simulink model "trzzy_kanaly_serial_real"  (R2025b)
settings: Solver=VariableStepAuto  StartTime=0.0  StopTime=0.5  RelTol=1e-3
undefined symbols (not defined in the file or in its folder): c, dspblkCoreblockFVToolHelper, gcbh, sfvc784, xck26
libraries: hdlBasic x68, simulink x5, hdlUtilities x4, vmcUtilities x1
settings Model: Creator=janek  LastModifiedBy=janek

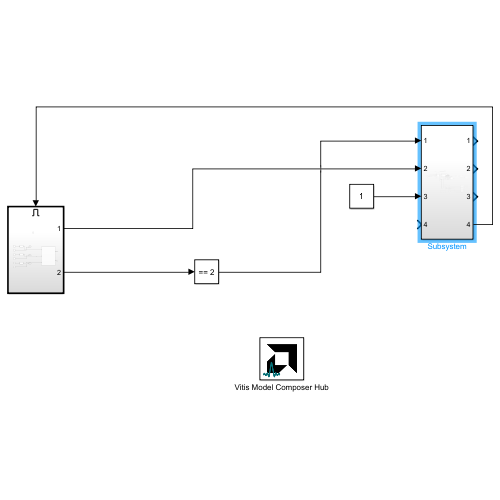
[thumbnail: Simulink's stored preview of the top-level diagram]
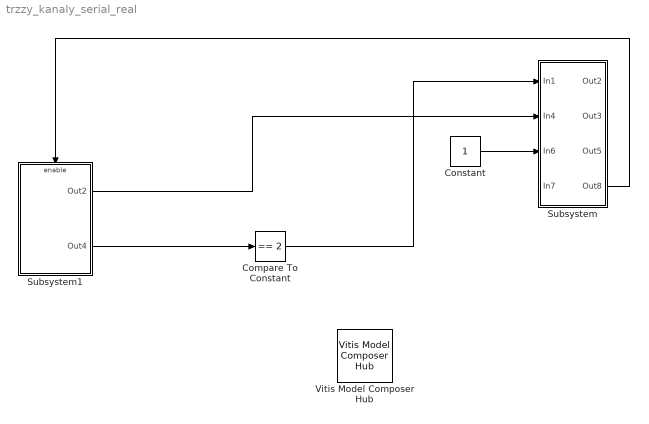
== system trzzy_kanaly_serial_real ==
  Compare To Constant : simulink/Logic and Bit Operations/Compare To Constant  relop===  const=2  OutDataTypeStr=boolean
  Constant : Constant
  Subsystem : Subsystem
  Subsystem1 : Subsystem
  Vitis Model Composer Hub : vmcUtilities/Vitis Model Composer Hub  Tag=genX  CodeGeneration=off  SubsystemName=Subsystem  CompilationType=HDLCompilation  ExportTypeV2=IP Catalog  StartColumn=1  NumberOfColumns=1  TargetDirectory=./netlist  exportDesign=off  analyzeDesign=off  validateDesignOnHw=off  ExportType=AI Engines  IpVendor=xilinx.com  IpLibrary=hls  IpVersion=1.0  IpHWLanguage=Verilog  AieCompilerOptions={}  AieSimulatorOptions={}  CreateTestbench=off  TestbenchStackSize=10  RunRtlSim=off  RunCSim=off  RunAieSim=off  AieSimTimeout=50000  RunAieSimProfiling=off  LaunchVitisAnalyzer=off  PlotOutput=off  RunX86Sim=off  X86SimTimeout=10  GenHwImage=off  GenLibadfXo=on  GenHwValidationCode=off  PlatformType=Not Specified  HwSystemType=Baremetal  HwValidationTarget=hw  ProjDevice=Kria KR260 Robotics Starter Kit SOM (xck26-sfvc784-2LV-c)  ProjDevicePart=xck26-sfvc784-2LV-c  AIEType=None  SamplePeriod=-1  ClockFrequency=200  DataPathParallelism=1  xilinxfamily=zynquplus  part=xck26  speed=-2LV-c  package=sfvc784  directory=./netlist\ip\Subsystem\src  testbench=off  incr_netlist=off  synthesis_tool=Vivado  clock_wrapper=Clock Enables  dbl_ovrd=According to Block Masks  dcm_input_clock_period=10  sysclk_period=40  simulink_period=1/81000  eval_field=0  LogFileName=''  NThreads=4
  wires:
  Compare To Constant/1 -> Subsystem/1(In1)
  Constant/1 -> Subsystem/3(In6)
  Subsystem1/2(Out4) -> Compare To Constant/1
  Subsystem/4(Out8) -> Subsystem1/Enable
  Subsystem1/1(Out2) -> Subsystem/2(In4)

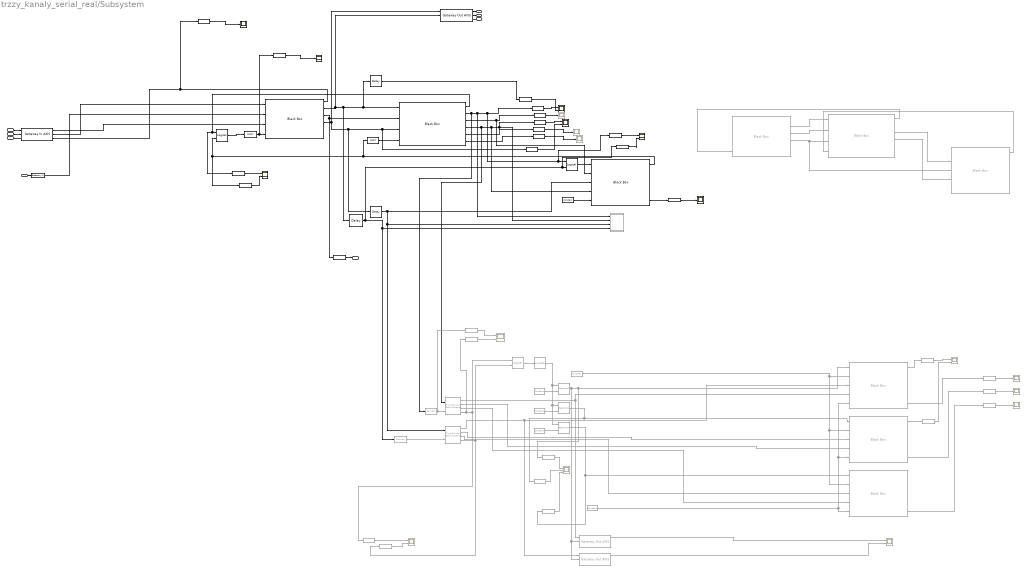
== system trzzy_kanaly_serial_real/Subsystem ==
  In1 : Inport
  In4 : Inport  Port=2
  In6 : Inport  Port=3
  In7 : Inport  Port=4
  Assert : hdlBasic/Assert  assert_type=on  type_source=Explicitly  gui_display_data_type=Fixed-point  arith_type=Unsigned  n_bits=1  bin_pt=0  preci_type=Single  exp_width=8  frac_width=24  assert_rate=on  rate_source=Explicitly  period=1/81000  output_port=on  XmcBlockStatus=1  maskContainerNames=group1  block_type=assert  block_config=sysgen:assert_config  block_width=609  block_height=900
  Assert1 : hdlBasic/Assert  assert_type=on  type_source=Explicitly  gui_display_data_type=Fixed-point  arith_type=Unsigned  n_bits=1  bin_pt=0  preci_type=Single  exp_width=8  frac_width=24  assert_rate=on  rate_source=Explicitly  period=1/81000  output_port=on  XmcBlockStatus=1  maskContainerNames=group1  block_type=assert  block_config=sysgen:assert_config  block_width=609  block_height=900
  Black Box : hdlBasic/Black Box  init_code=fir_compiler_0_wrapper_config  sim_method=Vivado Simulator  verbose=off  XmcBlockStatus=1  maskContainerNames=group1  block_type=blackbox2  block_config=sysgen:black_box_config
  Black Box1 : hdlBasic/Black Box  init_code=fir_compiler_1_wrapper_config  sim_method=Vivado Simulator  verbose=off  XmcBlockStatus=1  maskContainerNames=group1  block_type=blackbox2  block_config=sysgen:black_box_config
  Black Box2 : hdlBasic/Black Box  Commented=on  init_code=fir_compiler_0_wrapper_config  sim_method=Vivado Simulator  verbose=off  XmcBlockStatus=1  maskContainerNames=group1  block_type=blackbox2  block_config=sysgen:black_box_config
  Black Box3 : hdlBasic/Black Box  Commented=on  init_code=fir_compiler_1_wrapper_config  sim_method=Vivado Simulator  verbose=off  XmcBlockStatus=1  maskContainerNames=group1  block_type=blackbox2  block_config=sysgen:black_box_config
  Black Box{4,7..9} (4 alike) : hdlBasic/Black Box  Commented=on  init_code=cordic_0_wrapper_config  sim_method=Vivado Simulator  verbose=off  XmcBlockStatus=1  maskContainerNames=group1  block_type=blackbox2  block_config=sysgen:black_box_config
  Black Box5 : hdlBasic/Black Box  init_code=cordic_0_wrapper_config  sim_method=Vivado Simulator  verbose=off  XmcBlockStatus=1  maskContainerNames=group1  block_type=blackbox2  block_config=sysgen:black_box_config
  Constant : hdlBasic/Constant  const=1.0  gui_display_data_type=Boolean  arith_type=Boolean  n_bits=16  bin_pt=14  preci_type=Single  exp_width=8  frac_width=24  explicit_period=off  period=1  XmcBlockStatus=1  maskContainerNames=tabcontainer1  block_type=constant  block_config=sysgen:Constant_config
  Constant3 : hdlBasic/Constant  Commented=on  const=0  gui_display_data_type=Fixed-point  arith_type=Signed (2's comp)  n_bits=2  bin_pt=0  preci_type=Single  exp_width=8  frac_width=24  explicit_period=off  period=1  XmcBlockStatus=1  maskContainerNames=tabcontainer1  block_type=constant  block_config=sysgen:Constant_config
  Constant4 : hdlBasic/Constant  Commented=on  const=1.0  gui_display_data_type=Fixed-point  arith_type=Unsigned  n_bits=2  bin_pt=0  preci_type=Single  exp_width=8  frac_width=24  explicit_period=off  period=1  XmcBlockStatus=1  maskContainerNames=tabcontainer1  block_type=constant  block_config=sysgen:Constant_config
  Constant5 : hdlBasic/Constant  Commented=on  const=2  gui_display_data_type=Fixed-point  arith_type=Unsigned  n_bits=2  bin_pt=0  preci_type=Single  exp_width=8  frac_width=24  explicit_period=off  period=1  XmcBlockStatus=1  maskContainerNames=tabcontainer1  block_type=constant  block_config=sysgen:Constant_config
  Constant6 : hdlBasic/Constant  Commented=on  const=1.0  gui_display_data_type=Boolean  arith_type=Boolean  n_bits=16  bin_pt=14  preci_type=Single  exp_width=8  frac_width=24  explicit_period=off  period=1  XmcBlockStatus=1  maskContainerNames=tabcontainer1  block_type=constant  block_config=sysgen:Constant_config
  Constant7 : hdlBasic/Constant  Commented=on  const=0  gui_display_data_type=Boolean  arith_type=Boolean  n_bits=2  bin_pt=0  preci_type=Single  exp_width=8  frac_width=24  explicit_period=off  period=1  XmcBlockStatus=1  maskContainerNames=tabcontainer1  block_type=constant  block_config=sysgen:Constant_config
  Convert5 : hdlBasic/Convert  Commented=on  gui_display_data_type=Boolean  arith_type=Boolean  n_bits=16  bin_pt=14  float_type=Single  exp_bits=8  fraction_bits=24  quantization=Truncate  overflow=Wrap  en=off  latency=0  pipeline=off  XmcBlockStatus=1  maskContainerNames=group2  block_type=convert  block_config=sysgen:Convert_config  block_width=595  block_height=885
  Convert6 : hdlBasic/Convert  Commented=on  gui_display_data_type=Boolean  arith_type=Boolean  n_bits=16  bin_pt=14  float_type=Single  exp_bits=8  fraction_bits=24  quantization=Truncate  overflow=Wrap  en=off  latency=0  pipeline=off  XmcBlockStatus=1  maskContainerNames=group2  block_type=convert  block_config=sysgen:Convert_config  block_width=595  block_height=885
  Counter : hdlBasic/Counter  Commented=on  cnt_type=Count limited  cnt_to=2  operation=Up  start_count=0  cnt_by_val=1  arith_type=Unsigned  n_bits=2  bin_pt=0  load_pin=off  rst=off  en=on  explicit_period=Explicit  period=1/27000  use_behavioral_HDL=off  implementation=Fabric  XmcBlockStatus=1  maskContainerNames=group1  block_type=counter  block_config=sysgen:Counter_config  block_width=531  block_height=1023
  Delay : hdlBasic/Delay  rst=off  en=off  latency=30  reg_retiming=off  XmcBlockStatus=1  maskContainerNames=group1  block_type=delay  block_config=sysgen:Delay_config
  Delay1 : hdlBasic/Delay  rst=off  en=off  latency=30  reg_retiming=off  XmcBlockStatus=1  maskContainerNames=group1  block_type=delay  block_config=sysgen:Delay_config
  Delay2 : hdlBasic/Delay  rst=off  en=off  latency=30  reg_retiming=off  XmcBlockStatus=1  maskContainerNames=group1  block_type=delay  block_config=sysgen:Delay_config
  Gateway In : hdlBasic/Gateway In  gui_display_data_type=Boolean  arith_type=Boolean  n_bits=16  bin_pt=14  preci_type=Single  exp_width=8  frac_width=24  rows=1  columns=1  quantization="Round  (unbiased: +/- Inf)"  overflow=Saturate  period=1/81000  UseAsADC=off  ADCChannel='1'  interface=None  automatic_assignment=on  address_offset=hex2dec('00')  intf_name=''  intf_description=''  default_value=0  timing_constraint=None  locs_specified=off  LOCs={}  io_standard={}  inherit_from_input=off  hdl_port=on  XmcBlockStatus=1  maskContainerNames=group4  block_type=gatewayin  block_config=sysgen:gateway_in_config  block_width_w=590  block_height_w=620  block_width=640  block_height=850
  Gateway In AXIS : hdlUtilities/Gateway In AXIS  gui_display_data_type=Fixed-point  arith_type=Signed (2's comp)  n_bits=16  bin_pt=14  preci_type=Custom  exp_width=16  frac_width=24  quantization="Round  (unbiased: +/- Inf)"  overflow=Wrap  bool_to_boolean=off  OutSampleTime=1/81000  block_type=gatewayinaxi  XmcBlockStatus=1
  Gateway Out{,1..14} (15 alike) : hdlBasic/Gateway Out  inherit_from_input=off  bool_to_boolean=off  hdl_port=on  rows=1  columns=1  UseAsDAC=off  DACChannel='1'  interface=None  automatic_assignment=on  address_offset=hex2dec('00')  intf_name=''  intf_description=''  timing_constraint=None  locs_specified=off  LOCs={}  io_standard={}  XmcBlockStatus=1  maskContainerNames=group4  block_type=gatewayout  block_config=sysgen:gateway_out_config  block_width_w=590  block_height_w=620  block_width=620  block_height=750
  Gateway Out AXIS : hdlUtilities/Gateway Out AXIS  mask_sample_period=1/81000  bool_to_boolean=off  block_type=gatewayoutaxi
  Gateway Out AXIS1 : hdlUtilities/Gateway Out AXIS  Commented=on  mask_sample_period=1/27000  bool_to_boolean=off  block_type=gatewayoutaxi
  Gateway Out AXIS2 : hdlUtilities/Gateway Out AXIS  Commented=on  mask_sample_period=1/27000  bool_to_boolean=off  block_type=gatewayoutaxi
  Gateway Out{18..29} (12 alike) : hdlBasic/Gateway Out  Commented=on  inherit_from_input=off  bool_to_boolean=off  hdl_port=on  rows=1  columns=1  UseAsDAC=off  DACChannel='1'  interface=None  automatic_assignment=on  address_offset=hex2dec('00')  intf_name=''  intf_description=''  timing_constraint=None  locs_specified=off  LOCs={}  io_standard={}  XmcBlockStatus=1  maskContainerNames=group4  block_type=gatewayout  block_config=sysgen:gateway_out_config  block_width_w=590  block_height_w=620  block_width=620  block_height=750
  Logical : hdlBasic/Logical  logical_function=AND  inputs=2  en=off  latency=0  precision=Full  arith_type=Unsigned  n_bits=16  bin_pt=0  align_bp=on  overflow=[]  quantization=[]  XmcBlockStatus=1  maskContainerNames=tabcontainer1  block_type=logical  block_config=sysgen:Logical_config
  Logical1 : hdlBasic/Logical  logical_function=AND  inputs=2  en=off  latency=0  precision=Full  arith_type=Unsigned  n_bits=16  bin_pt=0  align_bp=on  overflow=[]  quantization=[]  XmcBlockStatus=1  maskContainerNames=tabcontainer1  block_type=logical  block_config=sysgen:Logical_config
  Logical2 : hdlBasic/Logical  Commented=on  logical_function=AND  inputs=2  en=off  latency=0  precision=Full  arith_type=Unsigned  n_bits=16  bin_pt=0  align_bp=on  overflow=[]  quantization=[]  XmcBlockStatus=1  maskContainerNames=tabcontainer1  block_type=logical  block_config=sysgen:Logical_config
  Relational : hdlBasic/Relational  Commented=on  mode=a=b  op_type=Bool  en=off  latency=0  XmcBlockStatus=1  maskContainerNames=tabcontainer1  block_type=relational  block_config=sysgen:Relational_config
  Relational1 : hdlBasic/Relational  Commented=on  mode=a=b  op_type=Bool  en=off  latency=0  XmcBlockStatus=1  maskContainerNames=tabcontainer1  block_type=relational  block_config=sysgen:Relational_config
  Relational2 : hdlBasic/Relational  Commented=on  mode=a=b  op_type=Bool  en=off  latency=0  XmcBlockStatus=1  maskContainerNames=tabcontainer1  block_type=relational  block_config=sysgen:Relational_config
  Scope{,1,6..7} (4 alike) : Scope  NumInputPorts=2
      Scope settings: ActiveDisplayYMinimum=-0.12499999999999997  ActiveDisplayYMaximum=1.125
      Scope1 settings: ActiveDisplayYMinimum=-1  ActiveDisplayYMaximum=1
      Scope6 settings: ActiveDisplayYMinimum=-0.12499999999999997  ActiveDisplayYMaximum=1.125  DataLoggingVariableName=ScopeData6
      Scope7 settings: ActiveDisplayYMinimum=-0.12499999999999997  ActiveDisplayYMaximum=1.125  DataLoggingVariableName=ScopeData7
  Scope{2..4,15..17} (6 alike) : Scope  Commented=on
      Scope15 settings: ActiveDisplayYMinimum=-3.2137215999999993E+7  ActiveDisplayYMaximum=2.89234944E+8  DataLoggingVariableName=ScopeData15
      Scope16 settings: ActiveDisplayYMinimum=-3.2137215999999993E+7  ActiveDisplayYMaximum=2.89234944E+8  DataLoggingVariableName=ScopeData16
      Scope17 settings: ActiveDisplayYMinimum=-3.2137215999999993E+7  ActiveDisplayYMaximum=2.89234944E+8  DataLoggingVariableName=ScopeData17
      Scope2 settings: ActiveDisplayYMinimum=-1  ActiveDisplayYMaximum=1  DataLoggingVariableName=ScopeData2
      Scope3 settings: ActiveDisplayYMinimum=-1  ActiveDisplayYMaximum=1  DataLoggingVariableName=ScopeData3
      Scope4 settings: ActiveDisplayYMinimum=-0.12499999999999997  ActiveDisplayYMaximum=1.125  DataLoggingVariableName=ScopeData4
  Scope{18..21} (4 alike) : Scope  Commented=on  NumInputPorts=2
      Scope18 settings: ActiveDisplayYMinimum=-0.12499999999999997  ActiveDisplayYMaximum=1.125  DataLoggingVariableName=ScopeData18
      Scope19 settings: ActiveDisplayYMinimum=-0.12499999999999997  ActiveDisplayYMaximum=1.125  DataLoggingVariableName=ScopeData19
      Scope20 settings: ActiveDisplayYMinimum=-0.12499999999999997  ActiveDisplayYMaximum=1.125  DataLoggingVariableName=ScopeData20
      Scope21 settings: ActiveDisplayYMinimum=-1  ActiveDisplayYMaximum=1  DataLoggingVariableName=ScopeData21
  Scope22 : Scope  Commented=on  NumInputPorts=3
      settings: ActiveDisplayYMinimum=-0.060135553546065944  ActiveDisplayYMaximum=1.0736512945264969  DataLoggingVariableName=ScopeData22
  Scope5 : Scope
      settings: ActiveDisplayYMinimum=-3.2137215999999993E+7  ActiveDisplayYMaximum=2.89234944E+8  DataLoggingVariableName=ScopeData5
  Scope8 : Scope
      settings: ActiveDisplayYMinimum=-0.12499999999999997  ActiveDisplayYMaximum=1.125  DataLoggingVariableName=ScopeData8
  Scope9 : Scope
      settings: ActiveDisplayYMinimum=-0.12499999999999997  ActiveDisplayYMaximum=1.125  DataLoggingVariableName=ScopeData9
  Subsystem : Subsystem  Commented=on
  Time Division Demultiplexer1 : hdlBasic/Time Division Demultiplexer  Commented=on  frame_pattern=[1 1 1]  impl_style=Multiple Channel  vin=on  explicit_period=off  period=1  XmcBlockStatus=1  maskContainerNames=group2  block_type=tdd  block_config=sysgen:TDD_config
  Time Division Demultiplexer4 : hdlBasic/Time Division Demultiplexer  Commented=on  frame_pattern=[1 1 1]  impl_style=Multiple Channel  vin=on  explicit_period=off  period=1  XmcBlockStatus=1  maskContainerNames=group2  block_type=tdd  block_config=sysgen:TDD_config
  Out2 : Outport
  Out3 : Outport  Port=2
  Out5 : Outport  Port=3
  Out8 : Outport  Port=4
  wires:
  Gateway Out AXIS/2 -> Out5/1
  In7/1 -> Gateway Out AXIS/3
  Gateway Out AXIS/1 -> Out3/1
  In6/1 -> Gateway In AXIS/2
  Gateway Out/1 -> Out2/1
  Gateway In AXIS/3 -> Out8/1
  In4/1 -> Gateway In AXIS/1
  In1/1 -> Gateway In/1
  Gateway In/1 -> Black Box/2
  Black Box/1 -> Gateway Out13/1, Gateway In AXIS/3
  Gateway In AXIS/2 -> Black Box/1
  Black Box/2 -> Delay/1, Black Box1/1, Delay2/1, Gateway Out AXIS/2
  Black Box/3 -> Black Box1/2, Gateway Out/1
  Black Box/4 -> Gateway Out AXIS/1, Delay1/1, Gateway Out6/1, Black Box1/3
  Gateway Out5/1 -> Scope3/1
  Gateway Out4/1 -> Scope2/1
  Gateway Out3/1 -> Scope1/1
  Gateway Out2/1 -> Scope4/1
  Gateway Out1/1 -> Scope/1
  Gateway In AXIS/1 -> Black Box/3
  Black Box1/1 -> Logical/1, Gateway Out12/1
  Black Box1/2 -> Subsystem/1(In1), Gateway Out9/1, Logical1/1, Gateway Out1/1, Convert6/1
  Black Box1/3 -> Black Box5/2, Gateway Out2/1
  Black Box1/4 -> Time Division Demultiplexer1/1, Black Box5/4, Subsystem/2(In2), Gateway Out3/1
  Black Box1/5 -> Gateway Out4/1
  Black Box1/6 -> Gateway Out5/1
  Assert/1 -> Gateway Out14/1, Black Box/4
  Gateway Out6/1 -> Scope1/2
  Delay/1 -> Gateway Out8/1
  Delay1/1 -> Black Box5/3, Time Division Demultiplexer4/1, Subsystem/3(In3)
  Delay2/1 -> Gateway Out10/1, Logical1/2, Convert5/1, Subsystem/4(In4)
  Gateway Out8/1 -> Scope/2
  Black Box5/1 -> Logical/2, Gateway Out11/1, Assert1/1
  Convert6/1 -> Time Division Demultiplexer1/2, Gateway Out26/1
  Convert5/1 -> Time Division Demultiplexer4/2
  Gateway Out24/1 -> Scope18/2
  Gateway Out25/1 -> Scope18/1
  Time Division Demultiplexer1/4 -> Gateway Out23/1, Logical2/1, Gateway Out25/1
  Time Division Demultiplexer4/4 -> Logical2/2, Gateway Out24/1
  Logical2/1 -> Counter/1
  Constant4/1 -> Relational1/2
  Constant5/1 -> Relational2/2
  Constant3/1 -> Relational/2
  Counter/1 -> Relational2/1, Relational1/1, Relational/1
  Relational/1 -> Gateway Out AXIS2/2, Gateway Out AXIS1/2, Gateway Out27/1, Black Box7/1
  Relational1/1 -> Gateway Out28/1, Black Box8/1
  Relational2/1 -> Gateway Out29/1, Black Box9/1
  Time Division Demultiplexer4/1 -> Gateway Out AXIS2/1, Black Box7/3
  Time Division Demultiplexer1/1 -> Black Box7/4, Gateway Out AXIS1/1
  Time Division Demultiplexer1/2 -> Black Box8/4
  Time Division Demultiplexer4/2 -> Black Box8/3
  Time Division Demultiplexer1/3 -> Black Box9/4
  Time Division Demultiplexer4/3 -> Black Box9/3
  Constant6/1 -> Black Box9/5, Black Box7/5, Black Box8/5
  Gateway Out18/1 -> Scope15/1
  Gateway Out19/1 -> Scope16/1
  Gateway Out20/1 -> Scope17/1
  Black Box7/4 -> Gateway Out18/1
  Black Box8/4 -> Gateway Out19/1
  Black Box9/4 -> Gateway Out20/1
  Constant7/1 -> Black Box9/2, Black Box8/2, Black Box7/2
  Black Box7/1 -> Gateway Out21/1
  Gateway Out23/1 -> Scope20/2
  Gateway Out26/1 -> Scope20/1
  Gateway Out AXIS1/1 -> Scope21/1
  Gateway Out AXIS2/1 -> Scope21/2
  Gateway Out27/1 -> Scope22/1
  Gateway Out28/1 -> Scope22/2
  Gateway Out29/1 -> Scope22/3
  Black Box8/1 -> Gateway Out22/1
  Gateway Out21/1 -> Scope19/1
  Gateway Out22/1 -> Scope19/2
  Black Box2/4 -> Black Box3/3, Black Box4/3
  Black Box3/4 -> Black Box4/4
  Black Box2/3 -> Black Box3/2
  Black Box2/2 -> Black Box3/1
  Black Box3/1 -> Black Box2/4
  Black Box3/3 -> Black Box4/2
  Black Box4/1 -> Black Box3/4
  Logical/1 -> Assert/1
  Logical1/1 -> Black Box5/1
  Assert1/1 -> Black Box1/4
  Constant/1 -> Black Box5/5
  Gateway Out7/1 -> Scope5/1
  Black Box5/4 -> Gateway Out7/1
  Gateway Out9/1 -> Scope6/1
  Gateway Out10/1 -> Scope6/2
  Gateway Out12/1 -> Scope7/1
  Gateway Out11/1 -> Scope7/2
  Gateway Out13/1 -> Scope8/1
  Gateway Out14/1 -> Scope9/1

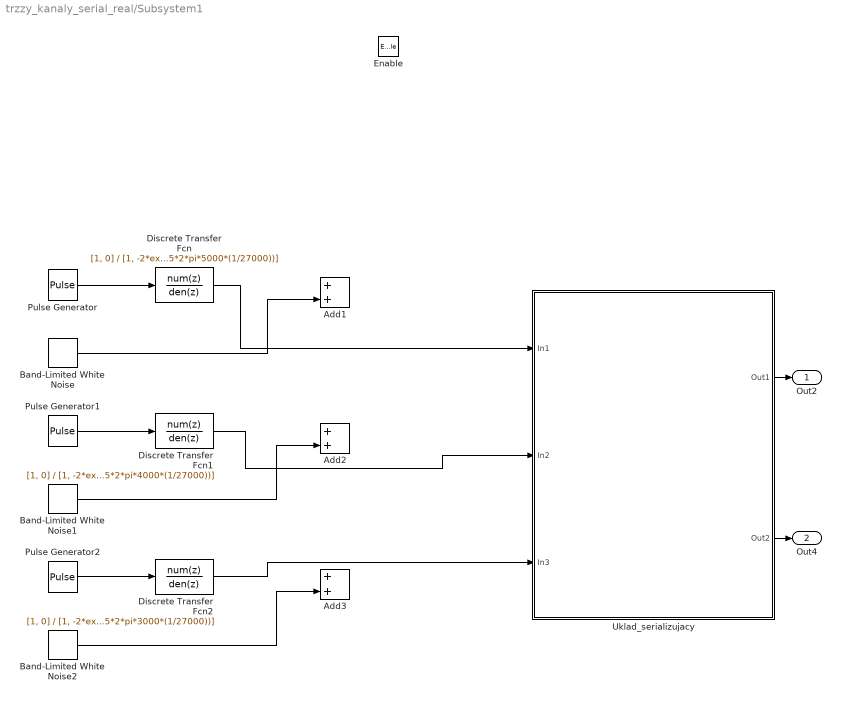
== system trzzy_kanaly_serial_real/Subsystem1 ==
  Enable : EnablePort
  Add1 : Sum
  Add2 : Sum
  Add3 : Sum
  Band-Limited White Noise : simulink/Sources/Band-Limited White Noise  Cov=[0.000001]  Ts=1/27000  seed=[23341]
  Band-Limited White Noise1 : simulink/Sources/Band-Limited White Noise  Cov=[0.000005]  Ts=1/27000  seed=[23341]
  Band-Limited White Noise2 : simulink/Sources/Band-Limited White Noise  Cov=[0.000005]  Ts=1/27000  seed=[23341]
  Discrete Transfer Fcn : DiscreteTransferFcn  LoadFcn=dspblkCoreblockFVToolHelper(gcbh,'load');  Numerator=[1, 0]  Denominator=[1, -2*exp(-0.05*2*pi*5000*(1/27000))*cos(2*pi*5000*sqrt(1-0.05^2)*(1/27000)), exp(-2*0.05*2*pi*5000*(1/27000))]
      settings: CopyFcn=dspblkCoreblockFVToolHelper(gcbh,'copy');  DeleteFcn=dspblkCoreblockFVToolHelper(gcbh,'close');  ModelCloseFcn=dspblkCoreblockFVToolHelper(gcbh,'close');  PreSaveFcn=dspblkCoreblockFVToolHelper(gcbh,'presave');  PostSaveFcn=dspblkCoreblockFVToolHelper(gcbh,'postsave');  CloseFcn=dspblkCoreblockFVToolHelper(gcbh,'close');
  Discrete Transfer Fcn1 : DiscreteTransferFcn  LoadFcn=dspblkCoreblockFVToolHelper(gcbh,'load');  Numerator=[1, 0]  Denominator=[1, -2*exp(-0.05*2*pi*5000*(1/27000))*cos(2*pi*4000*sqrt(1-0.05^2)*(1/27000)), exp(-2*0.05*2*pi*4000*(1/27000))]
      settings: CopyFcn=dspblkCoreblockFVToolHelper(gcbh,'copy');  DeleteFcn=dspblkCoreblockFVToolHelper(gcbh,'close');  ModelCloseFcn=dspblkCoreblockFVToolHelper(gcbh,'close');  PreSaveFcn=dspblkCoreblockFVToolHelper(gcbh,'presave');  PostSaveFcn=dspblkCoreblockFVToolHelper(gcbh,'postsave');  CloseFcn=dspblkCoreblockFVToolHelper(gcbh,'close');
  Discrete Transfer Fcn2 : DiscreteTransferFcn  LoadFcn=dspblkCoreblockFVToolHelper(gcbh,'load');  Numerator=[1, 0]  Denominator=[1, -2*exp(-0.05*2*pi*5000*(1/27000))*cos(2*pi*3000*sqrt(1-0.05^2)*(1/27000)), exp(-2*0.05*2*pi*3000*(1/27000))]
      settings: CopyFcn=dspblkCoreblockFVToolHelper(gcbh,'copy');  DeleteFcn=dspblkCoreblockFVToolHelper(gcbh,'close');  ModelCloseFcn=dspblkCoreblockFVToolHelper(gcbh,'close');  PreSaveFcn=dspblkCoreblockFVToolHelper(gcbh,'presave');  PostSaveFcn=dspblkCoreblockFVToolHelper(gcbh,'postsave');  CloseFcn=dspblkCoreblockFVToolHelper(gcbh,'close');
  Pulse Generator : DiscretePulseGenerator  Period=540  SampleTime=1/27000
  Pulse Generator1 : DiscretePulseGenerator  Period=675  SampleTime=1/27000
  Pulse Generator2 : DiscretePulseGenerator  Period=900  SampleTime=1/27000
  Uklad_serializujacy : Subsystem
  Out2 : Outport
  Out4 : Outport  Port=2
  wires:
  Pulse Generator1/1 -> Discrete Transfer Fcn1/1
  Discrete Transfer Fcn1/1 -> Uklad_serializujacy/2(In2)
  Pulse Generator2/1 -> Discrete Transfer Fcn2/1
  Uklad_serializujacy/1(Out1) -> Out2/1
  Discrete Transfer Fcn2/1 -> Uklad_serializujacy/3(In3)
  Band-Limited White Noise2/1 -> Add3/2
  Pulse Generator/1 -> Discrete Transfer Fcn/1
  Band-Limited White Noise1/1 -> Add2/2
  Band-Limited White Noise/1 -> Add1/2
  Discrete Transfer Fcn/1 -> Uklad_serializujacy/1(In1)
  Uklad_serializujacy/2(Out2) -> Out4/1

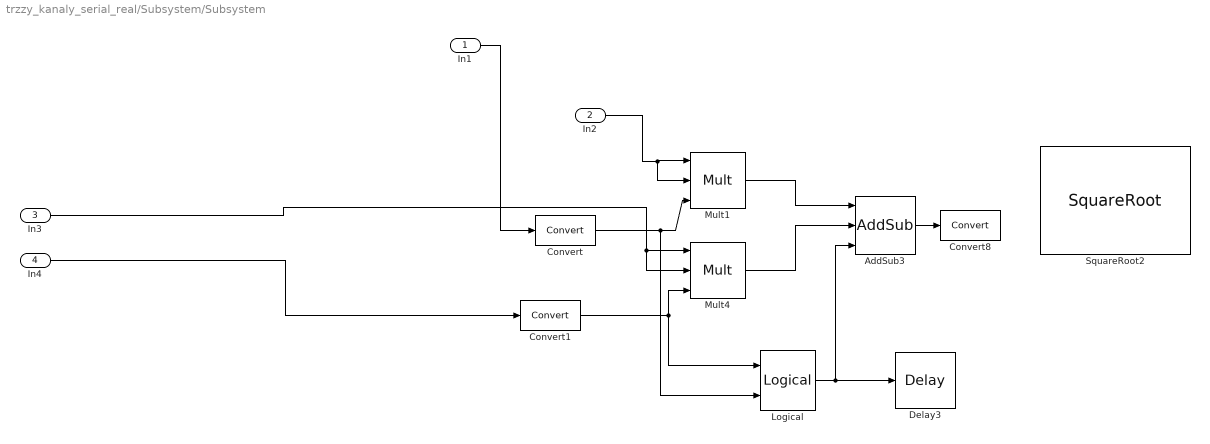
== system trzzy_kanaly_serial_real/Subsystem/Subsystem ==
  In1 : Inport
  In2 : Inport  Port=2
  In3 : Inport  Port=3
  In4 : Inport  Port=4
  AddSub3 : hdlBasic/AddSub  mode=Addition  use_carryin=off  use_carryout=off  en=on  latency=1  precision=Full  arith_type=Unsigned  n_bits=16  bin_pt=14  quantization=Truncate  overflow=Wrap  use_behavioral_HDL=off  hw_selection=Fabric  pipelined=off  XmcBlockStatus=1  maskContainerNames=tabcontainer1  block_type=addsub  block_config=sysgen:Addsub_config
  Convert : hdlBasic/Convert  gui_display_data_type=Boolean  arith_type=Boolean  n_bits=16  bin_pt=14  float_type=Single  exp_bits=8  fraction_bits=24  quantization=Truncate  overflow=Wrap  en=off  latency=0  pipeline=off  XmcBlockStatus=1  maskContainerNames=group2  block_type=convert  block_config=sysgen:Convert_config  block_width=595  block_height=885
  Convert1 : hdlBasic/Convert  gui_display_data_type=Boolean  arith_type=Boolean  n_bits=16  bin_pt=14  float_type=Single  exp_bits=8  fraction_bits=24  quantization=Truncate  overflow=Wrap  en=off  latency=0  pipeline=off  XmcBlockStatus=1  maskContainerNames=group2  block_type=convert  block_config=sysgen:Convert_config  block_width=595  block_height=885
  Convert8 : hdlBasic/Convert  gui_display_data_type=Floating-point  arith_type=Floating-point  n_bits=16  bin_pt=14  float_type=Single  exp_bits=8  fraction_bits=24  quantization="Round  (unbiased: +/- Inf)"  overflow=Saturate  en=off  latency=0  pipeline=off  XmcBlockStatus=1  maskContainerNames=group2  block_type=convert  block_config=sysgen:Convert_config  block_width=595  block_height=885
  Delay3 : hdlBasic/Delay  rst=off  en=off  latency=1  reg_retiming=off  XmcBlockStatus=1  maskContainerNames=group1  block_type=delay  block_config=sysgen:Delay_config
  Logical : hdlBasic/Logical  logical_function=AND  inputs=2  en=off  latency=1  precision=Full  arith_type=Unsigned  n_bits=16  bin_pt=0  align_bp=on  overflow=[]  quantization=[]  XmcBlockStatus=1  maskContainerNames=tabcontainer1  block_type=logical  block_config=sysgen:Logical_config
  Mult1 : hdlBasic/Mult  precision=User Defined  arith_type="Signed  (2's comp)"  n_bits=16  bin_pt=14  quantization="Round  (unbiased: +/- Inf)"  overflow=Saturate  en=on  latency=1  opt_float=off  fp_mult_usage=No Usage  use_behavioral_HDL=off  opt=Speed  use_embedded=on  optimum_pipeline=off  pipeline=on  use_rpm=on  placement_style=Triangular  XmcBlockStatus=1  maskContainerNames=group1  block_type=mult  block_config=sysgen:Mult_config  block_width=598  block_height=876
  Mult4 : hdlBasic/Mult  precision=User Defined  arith_type="Signed  (2's comp)"  n_bits=16  bin_pt=14  quantization="Round  (unbiased: +/- Inf)"  overflow=Saturate  en=on  latency=1  opt_float=off  fp_mult_usage=No Usage  use_behavioral_HDL=off  opt=Speed  use_embedded=on  optimum_pipeline=off  pipeline=on  use_rpm=on  placement_style=Triangular  XmcBlockStatus=1  maskContainerNames=group1  block_type=mult  block_config=sysgen:Mult_config  block_width=598  block_height=876
  SquareRoot2 : hdlBasic/SquareRoot  flow_control=Blocking  axi_optimize_goal=Resources  latency=1  rate=1  has_a_tlast=off  has_a_tuser=off  en=off  has_result_tready=on  has_invalid_op=off  fpo_op_type=square_root  has_b_tlast=false  has_b_tuser=false  result_tlast_behv=1  has_underflow=false  has_overflow=false  has_divide_by_zero=false  XmcBlockStatus=1  maskContainerNames=tabcontainer1  block_type=squareroot  block_config=sysgen:FPOBlockDescriptor_config
  wires:
  Mult4/1 -> AddSub3/2
  Convert/1 -> Logical/2, Mult1/3
  Convert1/1 -> Logical/1, Mult4/3
  In2/1 -> Mult1/2, Mult1/1
  Logical/1 -> Delay3/1, AddSub3/3
  AddSub3/1 -> Convert8/1
  Mult1/1 -> AddSub3/1
  In3/1 -> Mult4/2, Mult4/1
  In4/1 -> Convert1/1
  In1/1 -> Convert/1

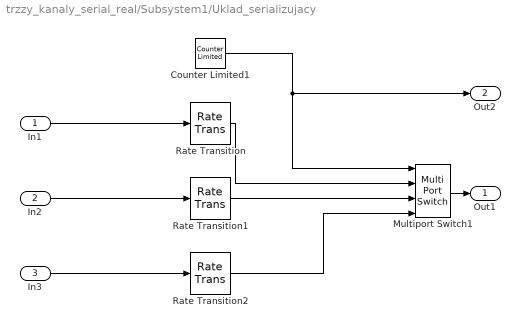
== system trzzy_kanaly_serial_real/Subsystem1/Uklad_serializujacy ==
  In1 : Inport
  In2 : Inport  Port=2
  In3 : Inport  Port=3
  Counter Limited1 : simulink/Sources/Counter Limited  uplimit=2  tsamp=1/81000
  Multiport Switch1 : MultiPortSwitch  DataPortOrder=Zero-based contiguous  zeroidx=on  SaturateOnIntegerOverflow=off  InputSameDT=off
  Rate Transition : RateTransition  OutPortSampleTime=1/81000
  Rate Transition1 : RateTransition  OutPortSampleTime=1/81000
  Rate Transition2 : RateTransition  OutPortSampleTime=1/81000
  Out1 : Outport
  Out2 : Outport  Port=2
  wires:
  In1/1 -> Rate Transition/1
  Rate Transition2/1 -> Multiport Switch1/4
  Counter Limited1/1 -> Out2/1, Multiport Switch1/1
  Rate Transition1/1 -> Multiport Switch1/3
  In2/1 -> Rate Transition1/1
  Rate Transition/1 -> Multiport Switch1/2
  In3/1 -> Rate Transition2/1
  Multiport Switch1/1 -> Out1/1
